simulink model "G3P3_System"  (R2020a)
settings: Solver=VariableStepAuto  StartTime=0.0  StopTime=10.0  RelTol=1e-3
settings Model: Creator=kadenplewe  LastModifiedBy=kadenplewe

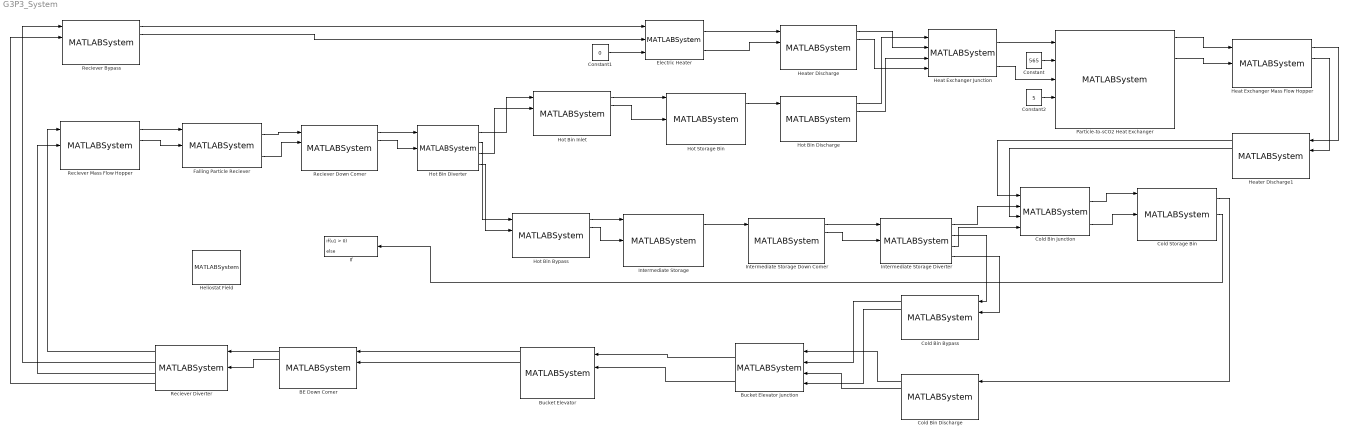
== system G3P3_System ==
  BE Down Comer : MATLABSystem  System=FFD  n=100  D=0.25  L=1  td=0.003  SimulateUsing=Code generation  Ts0=25  Tm0=25  cp_s=1250  rho_s=3500  phi_s=0.6  cp_m=500  rho_m=8000  hinf=10  hsw=100
      mask Type: FFD
      mask Display:
      | disp('FFD');
      | port_label('input',1,'Ts_in');
      | port_label('input',2,'mdot_s_in');
      | port_label('input',3,'Tinf');
      | port_label('input',4,'t');
      | port_label('output',1,'Ts_out');
      | port_label('output',2,'mdot_s_out');
      | port_label('output',3,'Ts');
      | port_label('output',4,'Tm');
      | port_label('output',5,'x');
  Bucket Elevator : MATLABSystem  System=BE  n=100  W=1  L=2  H=50  tm=0.006  SimulateUsing=Code generation  Ts0=25  Tm0=25  cp_s=1250  rho_s=3500  phi_s=0.6  cp_m=500  rho_m=8000  hinf=10  hsw=180
      mask Type: BE
      mask Display:
      | disp('BE');
      | port_label('input',1,'Ts_in');
      | port_label('input',2,'mdot_s_in');
      | port_label('input',3,'Tinf');
      | port_label('input',4,'t');
      | port_label('output',1,'Ts_out');
      | port_label('output',2,'mdot_s_out');
      | port_label('output',3,'Ts');
      | port_label('output',4,'Tm');
      | port_label('output',5,'x');
  Bucket Elevator Junction : MATLABSystem  System=SJ  cp_s=1250  Tref=0  SimulateUsing=Code generation
      mask Type: SJ
      mask Display:
      | disp('SJ');
      | port_label('input',1,'Ts_in1');
      | port_label('input',2,'Ts_in2');
      | port_label('input',3,'mdot_in1');
      | port_label('input',4,'mdot_in2');
      | port_label('output',1,'Ts_out');
      | port_label('output',2,'mdot_out');
  Cold Bin Bypass : MATLABSystem  System=FFD  n=100  D=0.25  L=1  td=0.003  SimulateUsing=Code generation  Ts0=25  Tm0=25  cp_s=1250  rho_s=3500  phi_s=0.6  cp_m=500  rho_m=8000  hinf=10  hsw=100
      mask Type: FFD
      mask Display:
      | disp('FFD');
      | port_label('input',1,'Ts_in');
      | port_label('input',2,'mdot_s_in');
      | port_label('input',3,'Tinf');
      | port_label('input',4,'t');
      | port_label('output',1,'Ts_out');
      | port_label('output',2,'mdot_s_out');
      | port_label('output',3,'Ts');
      | port_label('output',4,'Tm');
      | port_label('output',5,'x');
  Cold Bin Discharge : MATLABSystem  System=FFD  n=100  D=0.25  L=1  td=0.003  SimulateUsing=Code generation  Ts0=25  Tm0=25  cp_s=1250  rho_s=3500  phi_s=0.6  cp_m=500  rho_m=8000  hinf=10  hsw=100
      mask Type: FFD
      mask Display:
      | disp('FFD');
      | port_label('input',1,'Ts_in');
      | port_label('input',2,'mdot_s_in');
      | port_label('input',3,'Tinf');
      | port_label('input',4,'t');
      | port_label('output',1,'Ts_out');
      | port_label('output',2,'mdot_s_out');
      | port_label('output',3,'Ts');
      | port_label('output',4,'Tm');
      | port_label('output',5,'x');
  Cold Bin Junction : MATLABSystem  System=SJ  cp_s=1250  Tref=0  SimulateUsing=Code generation
      mask Type: SJ
      mask Display:
      | disp('SJ');
      | port_label('input',1,'Ts_in1');
      | port_label('input',2,'Ts_in2');
      | port_label('input',3,'mdot_in1');
      | port_label('input',4,'mdot_in2');
      | port_label('output',1,'Ts_out');
      | port_label('output',2,'mdot_out');
  Cold Storage Bin : MATLABSystem  System=LSB  H=1.5  D=2.4  SimulateUsing=Code generation  ms0=1  Ts0=615  ht=10  hinf=10  cp_s=1250  rho_s=3500  phi_s=0.6
      mask Type: LSB
      mask Display:
      | disp('LSB');
      | port_label('input',1,'Ts_in');
      | port_label('input',2,'Tinf');
      | port_label('input',3,'mdot_s_in');
      | port_label('input',4,'mdot_s_out');
      | port_label('input',5,'t');
      | port_label('output',1,'Ts_out');
      | port_label('output',2,'ms');
      | port_label('output',3,'qloss');
  Constant : Constant  Value=565
  Constant1 : Constant  Value=0
  Constant2 : Constant  Value=5
  Electric Heater : MATLABSystem  System=EH  cp_s=1250  SimulateUsing=Code generation
      mask Type: EH
      mask Display:
      | disp('EH');
      | port_label('input',1,'Ts_in');
      | port_label('input',2,'mdot_in');
      | port_label('input',3,'Qin');
      | port_label('output',1,'Ts_out');
      | port_label('output',2,'mdot_out');
  Falling Particle Reciever : MATLABSystem  System=FPR  H=1.2  W=1.2  d=0.0417  SimulateUsing=Code generation  Ts0=25  cp_s=1250  rho_s=3500  phi_s=0.6  epsilon_s=0.88  alpha_s=0.92
      mask Type: FPR
      mask Display:
      | disp('FPR');
      | port_label('input',1,'Ts_in');
      | port_label('input',2,'Tinf');
      | port_label('input',3,'mdot_s_in');
      | port_label('input',4,'Qsolar');
      | port_label('input',5,'t');
      | port_label('output',1,'Ts_out');
      | port_label('output',2,'mdot_s_out');
  Heat Exchanger Junction : MATLABSystem  System=SJ  cp_s=1250  Tref=0  SimulateUsing=Code generation
      mask Type: SJ
      mask Display:
      | disp('SJ');
      | port_label('input',1,'Ts_in1');
      | port_label('input',2,'Ts_in2');
      | port_label('input',3,'mdot_in1');
      | port_label('input',4,'mdot_in2');
      | port_label('output',1,'Ts_out');
      | port_label('output',2,'mdot_out');
  Heat Exchanger Mass Flow Hopper : MATLABSystem  System=MFH  n=20  H=1  D=1.2  SimulateUsing=Code generation  Ts0=25  cp_s=1250  rho_s=3500  phi_s=0.6
      mask Type: MFH
      mask Display:
      | disp('MFH');
      | port_label('input',1,'Ts_in');
      | port_label('input',2,'mdot_s_in');
      | port_label('input',3,'t');
      | port_label('output',1,'Ts_out');
      | port_label('output',2,'mdot_s_out');
      | port_label('output',3,'Ts');
      | port_label('output',4,'x');
  Heater Discharge : MATLABSystem  System=FFD  n=100  D=0.25  L=1  td=0.003  SimulateUsing=Code generation  Ts0=25  Tm0=25  cp_s=1250  rho_s=3500  phi_s=0.6  cp_m=500  rho_m=8000  hinf=10  hsw=100
      mask Type: FFD
      mask Display:
      | disp('FFD');
      | port_label('input',1,'Ts_in');
      | port_label('input',2,'mdot_s_in');
      | port_label('input',3,'Tinf');
      | port_label('input',4,'t');
      | port_label('output',1,'Ts_out');
      | port_label('output',2,'mdot_s_out');
      | port_label('output',3,'Ts');
      | port_label('output',4,'Tm');
      | port_label('output',5,'x');
  Heater Discharge1 : MATLABSystem  System=FFD  n=100  D=0.25  L=1  td=0.003  SimulateUsing=Code generation  Ts0=25  Tm0=25  cp_s=1250  rho_s=3500  phi_s=0.6  cp_m=500  rho_m=8000  hinf=10  hsw=100
      mask Type: FFD
      mask Display:
      | disp('FFD');
      | port_label('input',1,'Ts_in');
      | port_label('input',2,'mdot_s_in');
      | port_label('input',3,'Tinf');
      | port_label('input',4,'t');
      | port_label('output',1,'Ts_out');
      | port_label('output',2,'mdot_s_out');
      | port_label('output',3,'Ts');
      | port_label('output',4,'Tm');
      | port_label('output',5,'x');
  Heliostat Field : MATLABSystem  System=HF  n=150  H=5  W=5  eta_op=0.6  SimulateUsing=Code generation
      mask Type: HF
      mask Display:
      | disp('HF');
      | port_label('input',1,'DNI');
      | port_label('output',1,'Q_rec');
  Hot Bin Bypass : MATLABSystem  System=FFD  n=100  D=0.25  L=1  td=0.003  SimulateUsing=Code generation  Ts0=25  Tm0=25  cp_s=1250  rho_s=3500  phi_s=0.6  cp_m=500  rho_m=8000  hinf=10  hsw=100
      mask Type: FFD
      mask Display:
      | disp('FFD');
      | port_label('input',1,'Ts_in');
      | port_label('input',2,'mdot_s_in');
      | port_label('input',3,'Tinf');
      | port_label('input',4,'t');
      | port_label('output',1,'Ts_out');
      | port_label('output',2,'mdot_s_out');
      | port_label('output',3,'Ts');
      | port_label('output',4,'Tm');
      | port_label('output',5,'x');
  Hot Bin Discharge : MATLABSystem  System=FFD  n=100  D=0.25  L=1  td=0.003  SimulateUsing=Code generation  Ts0=25  Tm0=25  cp_s=1250  rho_s=3500  phi_s=0.6  cp_m=500  rho_m=8000  hinf=10  hsw=100
      mask Type: FFD
      mask Display:
      | disp('FFD');
      | port_label('input',1,'Ts_in');
      | port_label('input',2,'mdot_s_in');
      | port_label('input',3,'Tinf');
      | port_label('input',4,'t');
      | port_label('output',1,'Ts_out');
      | port_label('output',2,'mdot_s_out');
      | port_label('output',3,'Ts');
      | port_label('output',4,'Tm');
      | port_label('output',5,'x');
  Hot Bin Diverter : MATLABSystem  System=SS  SimulateUsing=Code generation
      mask Type: SS
      mask Display:
      | disp('SS');
      | port_label('input',1,'Ts_in');
      | port_label('input',2,'mdot_in');
      | port_label('input',3,'y1');
      | port_label('output',1,'Ts_out1');
      | port_label('output',2,'Ts_out2');
      | port_label('output',3,'mdot_out1');
      | port_label('output',4,'mdot_out2');
  Hot Bin Inlet : MATLABSystem  System=FFD  n=100  D=0.25  L=1  td=0.003  SimulateUsing=Code generation  Ts0=25  Tm0=25  cp_s=1250  rho_s=3500  phi_s=0.6  cp_m=500  rho_m=8000  hinf=10  hsw=100
      mask Type: FFD
      mask Display:
      | disp('FFD');
      | port_label('input',1,'Ts_in');
      | port_label('input',2,'mdot_s_in');
      | port_label('input',3,'Tinf');
      | port_label('input',4,'t');
      | port_label('output',1,'Ts_out');
      | port_label('output',2,'mdot_s_out');
      | port_label('output',3,'Ts');
      | port_label('output',4,'Tm');
      | port_label('output',5,'x');
  Hot Storage Bin : MATLABSystem  System=LSB  H=1.5  D=2.4  SimulateUsing=Code generation  ms0=1  Ts0=615  ht=10  hinf=10  cp_s=1250  rho_s=3500  phi_s=0.6
      mask Type: LSB
      mask Display:
      | disp('LSB');
      | port_label('input',1,'Ts_in');
      | port_label('input',2,'Tinf');
      | port_label('input',3,'mdot_s_in');
      | port_label('input',4,'mdot_s_out');
      | port_label('input',5,'t');
      | port_label('output',1,'Ts_out');
      | port_label('output',2,'ms');
      | port_label('output',3,'qloss');
  If : If
  Intermediate Storage : MATLABSystem  System=LSB  H=1.5  D=2.4  SimulateUsing=Code generation  ms0=1  Ts0=615  ht=10  hinf=10  cp_s=1250  rho_s=3500  phi_s=0.6
      mask Type: LSB
      mask Display:
      | disp('LSB');
      | port_label('input',1,'Ts_in');
      | port_label('input',2,'Tinf');
      | port_label('input',3,'mdot_s_in');
      | port_label('input',4,'mdot_s_out');
      | port_label('input',5,'t');
      | port_label('output',1,'Ts_out');
      | port_label('output',2,'ms');
      | port_label('output',3,'qloss');
  Intermediate Storage Diverter : MATLABSystem  System=SS  SimulateUsing=Code generation
      mask Type: SS
      mask Display:
      | disp('SS');
      | port_label('input',1,'Ts_in');
      | port_label('input',2,'mdot_in');
      | port_label('input',3,'y1');
      | port_label('output',1,'Ts_out1');
      | port_label('output',2,'Ts_out2');
      | port_label('output',3,'mdot_out1');
      | port_label('output',4,'mdot_out2');
  Intermediate Storage Down Comer : MATLABSystem  System=FFD  n=100  D=0.25  L=1  td=0.003  SimulateUsing=Code generation  Ts0=25  Tm0=25  cp_s=1250  rho_s=3500  phi_s=0.6  cp_m=500  rho_m=8000  hinf=10  hsw=100
      mask Type: FFD
      mask Display:
      | disp('FFD');
      | port_label('input',1,'Ts_in');
      | port_label('input',2,'mdot_s_in');
      | port_label('input',3,'Tinf');
      | port_label('input',4,'t');
      | port_label('output',1,'Ts_out');
      | port_label('output',2,'mdot_s_out');
      | port_label('output',3,'Ts');
      | port_label('output',4,'Tm');
      | port_label('output',5,'x');
  Particle-to-sCO2 Heat Exchanger : MATLABSystem  System=HX  n=20  t_s=0.003  t_CO2=0.001  t_m=0.003  H=1.5  W=0.6  N_plate=33  SimulateUsing=Code generation  h_s=450  h_CO2=3000  cp_s=1250  rho_s=3500  phi_s=0.6  cp_CO2=1250  rho_CO2=110  cp_m=500  rho_m=8000
      mask Type: HX
      mask Display:
      | disp('HX');
      | port_label('input',1,'Ts_in');
      | port_label('input',2,'Tco2_in');
      | port_label('input',3,'mdot_s_in');
      | port_label('input',4,'mdot_CO2_in');
      | port_label('input',5,'t');
      | port_label('output',1,'Ts_out');
      | port_label('output',2,'Tco2_out');
      | port_label('output',3,'mdot_s_out');
      | port_label('output',4,'mdot_CO2_out');
      | port_label('output',5,'Ts');
      | port_label('output',6,'Tco2');
      | port_label('output',7,'Tm');
      | port_label('output',8,'Q_CO2');
      | port_label('output',9,'x');
  Reciever Bypass : MATLABSystem  System=FFD  n=100  D=0.25  L=1  td=0.003  SimulateUsing=Code generation  Ts0=25  Tm0=25  cp_s=1250  rho_s=3500  phi_s=0.6  cp_m=500  rho_m=8000  hinf=10  hsw=100
      mask Type: FFD
      mask Display:
      | disp('FFD');
      | port_label('input',1,'Ts_in');
      | port_label('input',2,'mdot_s_in');
      | port_label('input',3,'Tinf');
      | port_label('input',4,'t');
      | port_label('output',1,'Ts_out');
      | port_label('output',2,'mdot_s_out');
      | port_label('output',3,'Ts');
      | port_label('output',4,'Tm');
      | port_label('output',5,'x');
  Reciever Diverter : MATLABSystem  System=SS  SimulateUsing=Code generation
      mask Type: SS
      mask Display:
      | disp('SS');
      | port_label('input',1,'Ts_in');
      | port_label('input',2,'mdot_in');
      | port_label('input',3,'y1');
      | port_label('output',1,'Ts_out1');
      | port_label('output',2,'Ts_out2');
      | port_label('output',3,'mdot_out1');
      | port_label('output',4,'mdot_out2');
  Reciever Down Comer : MATLABSystem  System=FFD  n=100  D=0.25  L=1  td=0.003  SimulateUsing=Code generation  Ts0=25  Tm0=25  cp_s=1250  rho_s=3500  phi_s=0.6  cp_m=500  rho_m=8000  hinf=10  hsw=100
      mask Type: FFD
      mask Display:
      | disp('FFD');
      | port_label('input',1,'Ts_in');
      | port_label('input',2,'mdot_s_in');
      | port_label('input',3,'Tinf');
      | port_label('input',4,'t');
      | port_label('output',1,'Ts_out');
      | port_label('output',2,'mdot_s_out');
      | port_label('output',3,'Ts');
      | port_label('output',4,'Tm');
      | port_label('output',5,'x');
  Reciever Mass Flow Hopper : MATLABSystem  System=MFH  n=20  H=1  D=1.2  SimulateUsing=Code generation  Ts0=25  cp_s=1250  rho_s=3500  phi_s=0.6
      mask Type: MFH
      mask Display:
      | disp('MFH');
      | port_label('input',1,'Ts_in');
      | port_label('input',2,'mdot_s_in');
      | port_label('input',3,'t');
      | port_label('output',1,'Ts_out');
      | port_label('output',2,'mdot_s_out');
      | port_label('output',3,'Ts');
      | port_label('output',4,'x');
  wires:
  Bucket Elevator/1 -> BE Down Comer/1
  Bucket Elevator/2 -> BE Down Comer/2
  BE Down Comer/1 -> Reciever Diverter/1
  BE Down Comer/2 -> Reciever Diverter/2
  Reciever Diverter/1 -> Reciever Mass Flow Hopper/1
  Reciever Diverter/3 -> Reciever Mass Flow Hopper/2
  Reciever Diverter/2 -> Reciever Bypass/1
  Reciever Diverter/4 -> Reciever Bypass/2
  Reciever Bypass/1 -> Electric Heater/1
  Reciever Bypass/2 -> Electric Heater/2
  Electric Heater/1 -> Heater Discharge/1
  Electric Heater/2 -> Heater Discharge/2
  Reciever Mass Flow Hopper/1 -> Falling Particle Reciever/1
  Reciever Mass Flow Hopper/2 -> Falling Particle Reciever/3
  Falling Particle Reciever/1 -> Reciever Down Comer/1
  Falling Particle Reciever/2 -> Reciever Down Comer/2
  Reciever Down Comer/1 -> Hot Bin Diverter/1
  Reciever Down Comer/2 -> Hot Bin Diverter/2
  Hot Bin Diverter/1 -> Hot Bin Inlet/1
  Hot Bin Diverter/3 -> Hot Bin Inlet/2
  Hot Bin Inlet/1 -> Hot Storage Bin/1
  Hot Bin Inlet/2 -> Hot Storage Bin/3
  Hot Bin Diverter/2 -> Hot Bin Bypass/1
  Hot Bin Diverter/4 -> Hot Bin Bypass/2
  Hot Bin Bypass/1 -> Intermediate Storage/1
  Hot Bin Bypass/2 -> Intermediate Storage/3
  Intermediate Storage/1 -> Intermediate Storage Down Comer/1
  Hot Storage Bin/1 -> Hot Bin Discharge/1
  Heater Discharge/1 -> Heat Exchanger Junction/2
  Heater Discharge/2 -> Heat Exchanger Junction/4
  Hot Bin Discharge/1 -> Heat Exchanger Junction/1
  Hot Bin Discharge/2 -> Heat Exchanger Junction/3
  Heat Exchanger Junction/1 -> Particle-to-sCO2 Heat Exchanger/1
  Heat Exchanger Junction/2 -> Particle-to-sCO2 Heat Exchanger/3
  Particle-to-sCO2 Heat Exchanger/1 -> Heat Exchanger Mass Flow Hopper/1
  Particle-to-sCO2 Heat Exchanger/3 -> Heat Exchanger Mass Flow Hopper/2
  Intermediate Storage Down Comer/1 -> Intermediate Storage Diverter/1
  Intermediate Storage Down Comer/2 -> Intermediate Storage Diverter/2
  Heat Exchanger Mass Flow Hopper/1 -> Heater Discharge1/1
  Heat Exchanger Mass Flow Hopper/2 -> Heater Discharge1/2
  Heater Discharge1/1 -> Cold Bin Junction/1
  Heater Discharge1/2 -> Cold Bin Junction/3
  Intermediate Storage Diverter/1 -> Cold Bin Junction/2
  Intermediate Storage Diverter/3 -> Cold Bin Junction/4
  Cold Bin Junction/1 -> Cold Storage Bin/1
  Cold Bin Junction/2 -> Cold Storage Bin/3
  Intermediate Storage Diverter/2 -> Cold Bin Bypass/1
  Intermediate Storage Diverter/4 -> Cold Bin Bypass/2
  Cold Storage Bin/1 -> Cold Bin Discharge/1
  Cold Bin Bypass/1 -> Bucket Elevator Junction/2
  Cold Bin Discharge/1 -> Bucket Elevator Junction/1
  Cold Bin Discharge/2 -> Bucket Elevator Junction/3
  Cold Bin Bypass/2 -> Bucket Elevator Junction/4
  Bucket Elevator Junction/1 -> Bucket Elevator/1
  Bucket Elevator Junction/2 -> Bucket Elevator/2
  Constant1/1 -> Electric Heater/3
  Constant/1 -> Particle-to-sCO2 Heat Exchanger/2
  Constant2/1 -> Particle-to-sCO2 Heat Exchanger/4
  Cold Storage Bin/2 -> If/1
